simulink model "VRFT_dataCollect_IPCopenloop_sin3p"  (R2015a)
settings: Solver=ode3  StartTime=0.0  StopTime=TMax  FixedStep=DT  MaxStep=DT  RelTol=1e-3
values from neighbouring files (symbols this model uses):
  amp_square = 0.8    [exe_VRFT_dataCollect.m]
  center_square = 0    [exe_VRFT_dataCollect.m]
  square_period = 100    [exe_VRFT_dataCollect.m]
undefined symbols (not defined in the file or in its folder): amp_omega1, amp_omega2, amp_omega4, Avgyop, DT, NDOF, NumOuts, omega1, omega2, omega4, OutList, q_init, qdot_init, strmatch
libraries: simulink x1
settings Model: Creator=Vinicius  LastModifiedBy=mauri
settings DataIOCC: SignalLoggingSaveFormat=ModelDataLogs  SaveOutput=off  SaveTime=off  SignalLoggingName=sigsOut
settings OptimizationCC: ExpressionDepthLimit=2147483647
settings DebuggingCC: SaveWithParameterizedLinksMsg=none  UnderspecifiedInitializationDetection=Classic  MergeDetectMultiDrivingBlocksExec=none  SignalResolutionControl=TryResolveAllWithWarning  MultiTaskDSMMsg=warning  MultiTaskCondExecSysMsg=none  StateNameClashWarn=warning
settings HardwareCC: TargetLongLongMode=on  TargetIntDivRoundTo=Zero  TargetEndianess=LittleEndian  TargetHWDeviceType=MATLAB Host  ProdEqTarget=off
settings GRTTargetCC: CombineOutputUpdateFcns=off  GRTInterface=on

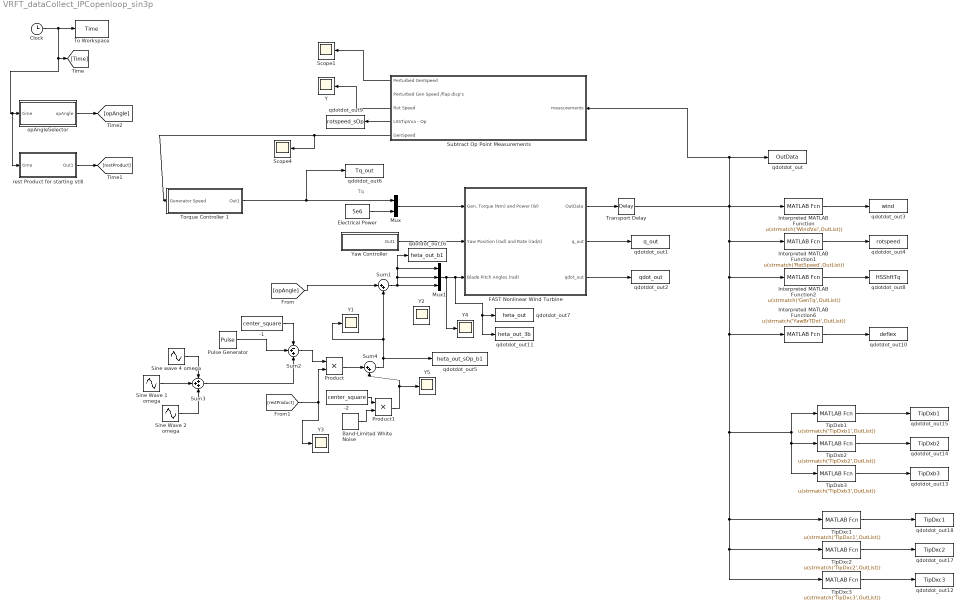
== system VRFT_dataCollect_IPCopenloop_sin3p ==
  note: Tq
  -1 : Constant  Value=center_square
  -2 : Constant  Value=center_square
  Band-Limited White Noise : simulink/Sources/Band-Limited White Noise  Cov=[1]  Ts=0.05  seed=[23341]
  Clock : Clock
  Electrical Power : Constant  Value=5e6
  FAST Nonlinear Wind Turbine : Subsystem  mask(FAST Nonlinear Wind Turbine){}
      mask help: This block contains the FAST S-Function and blocks that integrate the DOF accelerations to get velocities and displacements.
      mask init:
      | clear FAST_SFunc
  Interpreted MATLAB Function : MATLABFcn  MATLABFcn=u(strmatch('WindVxi',OutList))
  Interpreted MATLAB Function1 : MATLABFcn  MATLABFcn=u(strmatch('RotSpeed',OutList))
  Interpreted MATLAB Function2 : MATLABFcn  MATLABFcn=u(strmatch('GenTq',OutList))
  Interpreted MATLAB Function6 : MATLABFcn  MATLABFcn=u(strmatch('YawBrTDxt',OutList))
  Mux : Mux  Inputs=2
  Mux1 : Mux  Inputs=3
  Product : Product
  Product1 : Product
  Pulse Generator : DiscretePulseGenerator  PulseType=Time based  Amplitude=amp_square  Period=square_period  PulseWidth=50
  Scope1 : Scope
      settings: TimeRange=79.99800000000001  YMin=-52  YMax=-30
  Scope4 : Scope
      settings: TimeRange=79.99800000000001  YMin=190  YMax=350  SaveName=ScopeData2
  Sine Wave 1 omega : Sin  Amplitude=amp_omega1  Frequency=omega1  SampleTime=0
  Sine Wave 2 omega : Sin  Amplitude=amp_omega2  Frequency=omega2  SampleTime=0
  Sine wave 4 omega : Sin  Amplitude=amp_omega4  Frequency=omega4  SampleTime=0
  Subtract Op Point Measurements : Subsystem
  Sum1 : Sum  Inputs=|++
  Sum2 : Sum  Inputs=-++
  Sum3 : Sum  Inputs=+++
  Sum4 : Sum  Inputs=|++
  TipDxb1 : MATLABFcn  MATLABFcn=u(strmatch('TipDxb1',OutList))
  TipDxb2 : MATLABFcn  MATLABFcn=u(strmatch('TipDxb2',OutList))
  TipDxb3 : MATLABFcn  MATLABFcn=u(strmatch('TipDxb3',OutList))
  TipDxc1 : MATLABFcn  MATLABFcn=u(strmatch('TipDxc1',OutList))
  "TipDxc2 " : MATLABFcn  MATLABFcn=u(strmatch('TipDxc2',OutList))
  TipDxc3 : MATLABFcn  MATLABFcn=u(strmatch('TipDxc3',OutList))
  To Workspace : ToWorkspace  VariableName=Time  SampleTime=-1
  "Torque Controller 1 " : Subsystem
  Transport Delay : TransportDelay  DelayTime=1*DT
  Y{,1..5} (6 alike) : Scope
      Y settings: TimeRange=100  YMin=2.5  YMax=30  SaveName=ScopeData3
      Y1 settings: TimeRange=100  YMin=-0.0575  YMax=6.93889e-18
      Y2 settings: TimeRange=100  YMin=0.13  YMax=0.28  SaveName=ScopeData4
      Y3 settings: TimeRange=100  YMin=0.95  YMax=1.05  SaveName=ScopeData5
      Y4 settings: TimeRange=100  YMin=0.13  YMax=0.28  SaveName=ScopeData6
      Y5 settings: TimeRange=100  YMin=-0.0575  YMax=6.93889e-18  SaveName=ScopeData7
  Yaw Controller : Subsystem
  opAngleSelector : Subsystem
  qdotdot_out : ToWorkspace  VariableName=OutData  SampleTime=-1
  qdotdot_out1 : ToWorkspace  VariableName=q_out  SampleTime=-1
  qdotdot_out10 : ToWorkspace  VariableName=deflex  SampleTime=-1
  qdotdot_out11 : ToWorkspace  VariableName=heta_out_3b  SampleTime=-1
  qdotdot_out12 : ToWorkspace  VariableName=TipDxc3  SampleTime=-1
  qdotdot_out13 : ToWorkspace  VariableName=TipDxb3  SampleTime=-1
  qdotdot_out14 : ToWorkspace  VariableName=TipDxb2  SampleTime=-1
  qdotdot_out15 : ToWorkspace  VariableName=TipDxb1  SampleTime=-1
  qdotdot_out16 : ToWorkspace  VariableName=heta_out_b1  SampleTime=-1
  qdotdot_out17 : ToWorkspace  VariableName=TipDxc2  SampleTime=-1
  qdotdot_out18 : ToWorkspace  VariableName=TipDxc1  SampleTime=-1
  qdotdot_out2 : ToWorkspace  VariableName=qdot_out  SampleTime=-1
  qdotdot_out3 : ToWorkspace  VariableName=wind  SampleTime=-1
  qdotdot_out4 : ToWorkspace  VariableName=rotspeed  SampleTime=-1
  qdotdot_out5 : ToWorkspace  VariableName=heta_out_sOp_b1  SampleTime=-1
  qdotdot_out6 : ToWorkspace  VariableName=Tq_out  SampleTime=-1
  qdotdot_out7 : ToWorkspace  VariableName=heta_out  SampleTime=-1
  qdotdot_out8 : ToWorkspace  VariableName=HSShftTq  SampleTime=-1
  qdotdot_out9 : ToWorkspace  VariableName=rotspeed_sOp  SampleTime=-1
  rest Product for starting still : Subsystem
  wires:
  Clock/1 -> rest Product for starting still/1(time), opAngleSelector/1(time), [Time], To Workspace/1
  FAST Nonlinear Wind Turbine/2(q_out) -> qdotdot_out1/1
  FAST Nonlinear Wind Turbine/3(qdot_out) -> qdotdot_out2/1
  Yaw Controller/1(Out1) -> FAST Nonlinear Wind Turbine/2(Yaw Position (rad) and Rate (rad/s))
  Electrical Power/1 -> Mux/2
  FAST Nonlinear Wind Turbine/1(OutData) -> Transport Delay/1
  Interpreted MATLAB Function/1 -> qdotdot_out3/1
  Interpreted MATLAB Function1/1 -> qdotdot_out4/1
  Interpreted MATLAB Function2/1 -> qdotdot_out8/1
  Mux/1 -> FAST Nonlinear Wind Turbine/1(Gen. Torque (Nm) and Power (W))
  "Torque Controller 1 "/1(Out1) -> qdotdot_out6/1, Mux/1
  Subtract Op Point Measurements/5(GenSpeed) -> Scope4/1, "Torque Controller 1 "/1(Generator Speed)
  Subtract Op Point Measurements/1(Perturbed GenSpeed) -> Scope1/1
  Subtract Op Point Measurements/3(Rot Speed) -> Y/1
  Interpreted MATLAB Function6/1 -> qdotdot_out10/1
  [opAngle] -> Sum1/1
  Mux1/1 -> Y4/1, qdotdot_out11/1, qdotdot_out7/1, FAST Nonlinear Wind Turbine/3(Blade Pitch Angles (rad))
  -1/1 -> Sum2/1
  opAngleSelector/1("opAngle ") -> [opAngle]
  rest Product for starting still/1(Out1) -> [restProduct]
  [restProduct] -> Product/2, Y3/1
  Pulse Generator/1 -> Sum2/2
  Sum2/1 -> Product/1
  Subtract Op Point Measurements/4(LSSTipVxa - Op) -> qdotdot_out9/1
  Sum1/1 -> Mux1/2, qdotdot_out16/1, Mux1/1, Mux1/3
  TipDxb1/1 -> qdotdot_out15/1
  TipDxb3/1 -> qdotdot_out13/1
  TipDxb2/1 -> qdotdot_out14/1
  Transport Delay/1 -> Interpreted MATLAB Function/1, qdotdot_out/1, Subtract Op Point Measurements/1(measurements), TipDxc3/1, "TipDxc2 "/1, TipDxc1/1, TipDxb3/1, TipDxb2/1, TipDxb1/1, Interpreted MATLAB Function6/1, Interpreted MATLAB Function2/1, Interpreted MATLAB Function1/1
  TipDxc1/1 -> qdotdot_out18/1
  TipDxc3/1 -> qdotdot_out12/1
  "TipDxc2 "/1 -> qdotdot_out17/1
  Sine Wave 1 omega/1 -> Sum3/2
  Sine wave 4 omega/1 -> Sum3/1
  Sine Wave 2 omega/1 -> Sum3/3
  Sum3/1 -> Sum2/3
  Band-Limited White Noise/1 -> Product1/2
  -2/1 -> Product1/1
  Product1/1 -> Y5/1, Sum4/2
  Product/1 -> Sum4/1
  Sum4/1 -> Sum1/2, Y1/1, qdotdot_out5/1

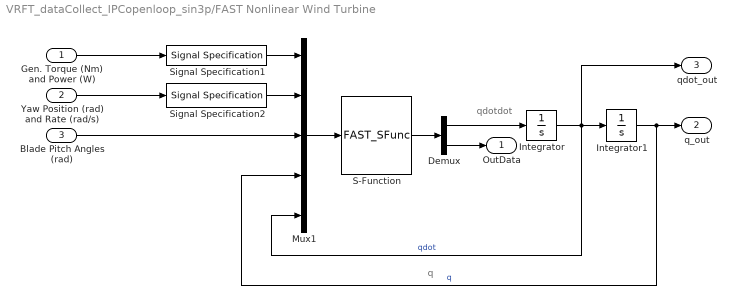
== system VRFT_dataCollect_IPCopenloop_sin3p/FAST Nonlinear Wind Turbine ==
  note: qdotdot
  note: q
  Gen. Torque (Nm) and Power (W) : Inport
  Yaw Position (rad) and Rate (rad/s) : Inport  Port=2
  Blade Pitch Angles (rad) : Inport  Port=3
  Demux : Demux  Outputs=[NDOF, NumOuts]
  Integrator : Integrator  InitialCondition=qdot_init
  Integrator1 : Integrator  InitialCondition=q_init
  Mux1 : Mux  Inputs=5
  S-Function : S-Function  FunctionName=FAST_SFunc
  Signal Specification1 : SignalSpecification  OutDataTypeStr=double  Dimensions=2
  Signal Specification2 : SignalSpecification  OutDataTypeStr=double  Dimensions=2
  OutData : Outport
  q_out : Outport  Port=2
  qdot_out : Outport  Port=3
  wires:
  Integrator/1 -> Mux1/5, qdot_out/1, Integrator1/1  "qdot"
  Gen. Torque (Nm) and Power (W)/1 -> Signal Specification1/1
  S-Function/1 -> Demux/1
  Demux/1 -> Integrator/1
  Demux/2 -> OutData/1
  Mux1/1 -> S-Function/1
  Blade Pitch Angles (rad)/1 -> Mux1/3
  Yaw Position (rad) and Rate (rad/s)/1 -> Signal Specification2/1
  Integrator1/1 -> q_out/1, Mux1/4  "q"
  Signal Specification1/1 -> Mux1/1
  Signal Specification2/1 -> Mux1/2

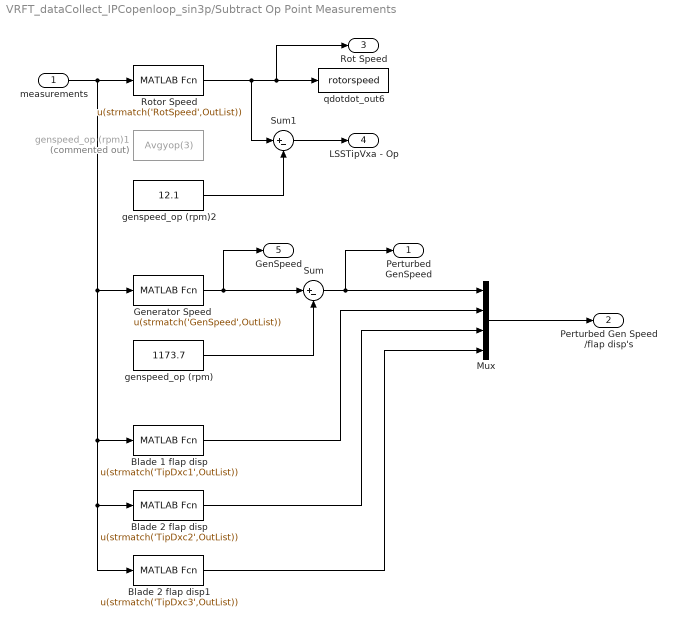
== system VRFT_dataCollect_IPCopenloop_sin3p/Subtract Op Point Measurements ==
  measurements : Inport
  Blade 1 flap disp : MATLABFcn  MATLABFcn=u(strmatch('TipDxc1',OutList))
  Blade 2 flap disp : MATLABFcn  MATLABFcn=u(strmatch('TipDxc2',OutList))
  Blade 2 flap disp1 : MATLABFcn  MATLABFcn=u(strmatch('TipDxc3',OutList))
  Generator Speed : MATLABFcn  MATLABFcn=u(strmatch('GenSpeed',OutList))
  Mux : Mux
  Rotor Speed : MATLABFcn  MATLABFcn=u(strmatch('RotSpeed',OutList))
  Sum : Sum  Inputs=|+-
  Sum1 : Sum  Inputs=|+-
  genspeed_op (rpm) : Constant  Value=1173.7
  genspeed_op (rpm)1 : Constant  Commented=on  Value=Avgyop(3)
  genspeed_op (rpm)2 : Constant  Value=12.1
  qdotdot_out6 : ToWorkspace  VariableName=rotorspeed  SampleTime=-1
  Perturbed GenSpeed : Outport
  Perturbed Gen Speed /flap disp's : Outport  Port=2
  Rot Speed : Outport  Port=3
  LSSTipVxa - Op : Outport  Port=4
  GenSpeed : Outport  Port=5
  wires:
  Rotor Speed/1 -> Sum1/1, Rot Speed/1, qdotdot_out6/1
  Sum/1 -> Perturbed GenSpeed/1, Mux/1
  Blade 1 flap disp/1 -> Mux/2
  Blade 2 flap disp/1 -> Mux/3
  Blade 2 flap disp1/1 -> Mux/4
  measurements/1 -> Blade 2 flap disp/1, Blade 2 flap disp1/1, Blade 1 flap disp/1, Generator Speed/1, Rotor Speed/1
  genspeed_op (rpm)/1 -> Sum/2
  Generator Speed/1 -> GenSpeed/1, Sum/1
  Mux/1 -> Perturbed Gen Speed /flap disp's/1
  Sum1/1 -> LSSTipVxa - Op/1
  genspeed_op (rpm)2/1 -> Sum1/2

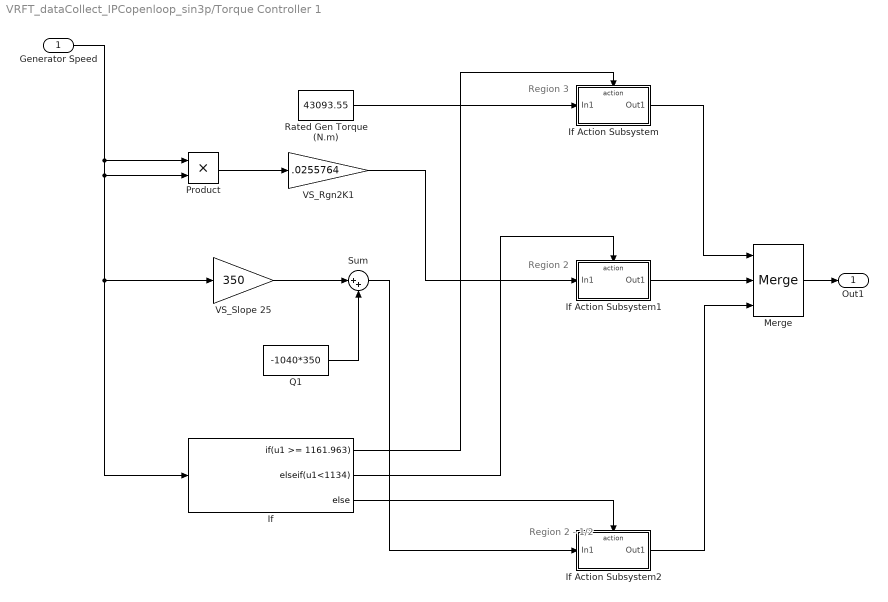
== system VRFT_dataCollect_IPCopenloop_sin3p/Torque Controller 1  ==
  note: Region 2 - 1/2
  note: Region 2
  note: Region 3
  Generator Speed : Inport
  If : If  IfExpression=u1 >= 1161.963  ElseIfExpressions=u1<1134
  If Action Subsystem : Subsystem  TreatAsAtomicUnit=on
  If Action Subsystem1 : Subsystem  TreatAsAtomicUnit=on
  If Action Subsystem2 : Subsystem  TreatAsAtomicUnit=on
  Merge : Merge  Inputs=3
  Product : Product  RndMeth=Zero
  Q1 : Constant  Value=-1040*350
  Rated Gen Torque (N.m) : Constant  Value=43093.55
  Sum : Sum  Inputs=|++
  VS_Rgn2K1 : Gain  Gain=.0255764
  VS_Slope 25 : Gain  Gain=350
  Out1 : Outport
  wires:
  Rated Gen Torque (N.m)/1 -> If Action Subsystem/1(In1)
  If/1 -> If Action Subsystem/Action
  If/2 -> If Action Subsystem1/Action
  If/3 -> If Action Subsystem2/Action
  If Action Subsystem2/1(Out1) -> Merge/3
  If Action Subsystem1/1(Out1) -> Merge/2
  If Action Subsystem/1(Out1) -> Merge/1
  Merge/1 -> Out1/1
  Generator Speed/1 -> Product/1, Product/2, VS_Slope 25/1, If/1
  Product/1 -> VS_Rgn2K1/1
  Q1/1 -> Sum/2
  VS_Slope 25/1 -> Sum/1
  Sum/1 -> If Action Subsystem2/1(In1)
  VS_Rgn2K1/1 -> If Action Subsystem1/1(In1)

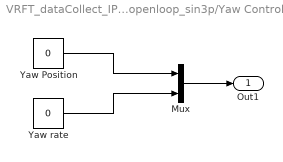
== system VRFT_dataCollect_IPCopenloop_sin3p/Yaw Controller ==
  Mux : Mux  Inputs=2
  Yaw Position : Constant  Value=0
  Yaw rate : Constant  Value=0
  Out1 : Outport
  wires:
  Mux/1 -> Out1/1
  Yaw Position/1 -> Mux/1
  Yaw rate/1 -> Mux/2

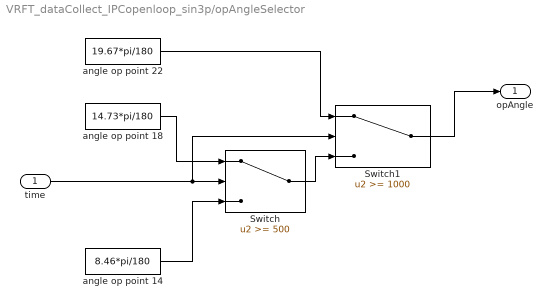
== system VRFT_dataCollect_IPCopenloop_sin3p/opAngleSelector ==
  time : Inport
  Switch : Switch  Threshold=500
  Switch1 : Switch  Threshold=1000
  angle op point 14 : Constant  Value=8.46*pi/180
  "angle op point 18 " : Constant  Value=14.73*pi/180
  angle op point 22 : Constant  Value=19.67*pi/180
  "opAngle " : Outport
  wires:
  angle op point 14/1 -> Switch/3
  Switch/1 -> Switch1/3
  "angle op point 18 "/1 -> Switch/1
  angle op point 22/1 -> Switch1/1
  Switch1/1 -> "opAngle "/1
  time/1 -> Switch1/2, Switch/2

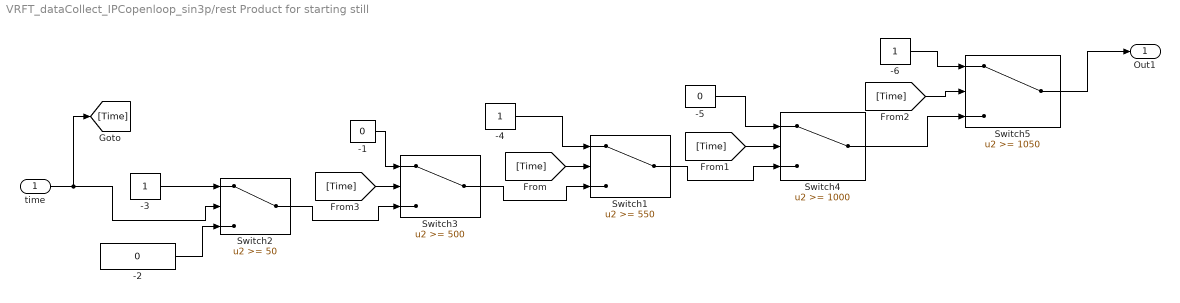
== system VRFT_dataCollect_IPCopenloop_sin3p/rest Product for starting still ==
  time : Inport
  -1 : Constant  Value=0
  -2 : Constant  Value=0
  -3 : Constant
  -4 : Constant
  -5 : Constant  Value=0
  -6 : Constant
  Switch1 : Switch  Threshold=550
  Switch2 : Switch  Threshold=50
  Switch3 : Switch  Threshold=500
  Switch4 : Switch  Threshold=1000
  Switch5 : Switch  Threshold=1050
  Out1 : Outport
  wires:
  -2/1 -> Switch2/3
  Switch2/1 -> Switch3/3
  -3/1 -> Switch2/1
  Switch3/1 -> Switch1/3
  Switch1/1 -> Switch4/3
  -1/1 -> Switch3/1
  -4/1 -> Switch1/1
  -5/1 -> Switch4/1
  -6/1 -> Switch5/1
  Switch4/1 -> Switch5/3
  Switch5/1 -> Out1/1
  time/1 -> [Time], Switch2/2
  [Time] -> Switch1/2
  [Time] -> Switch4/2
  [Time] -> Switch5/2
  [Time] -> Switch3/2

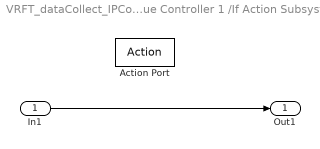
== system VRFT_dataCollect_IPCopenloop_sin3p/Torque Controller 1 /If Action Subsystem ==
  In1 : Inport
  Action Port : ActionPort  ActionType=then
  Out1 : Outport
  wires:
  In1/1 -> Out1/1

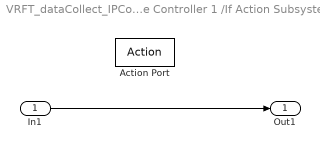
== system VRFT_dataCollect_IPCopenloop_sin3p/Torque Controller 1 /If Action Subsystem1 ==
  In1 : Inport
  Action Port : ActionPort  ActionType=elseif
  Out1 : Outport
  wires:
  In1/1 -> Out1/1

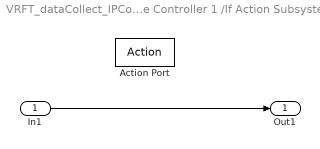
== system VRFT_dataCollect_IPCopenloop_sin3p/Torque Controller 1 /If Action Subsystem2 ==
  In1 : Inport
  Action Port : ActionPort  ActionType=else
  Out1 : Outport
  wires:
  In1/1 -> Out1/1
